simulink model "modelo_kibado_da_mathworks_que_n_funciona"  (R2023a)
settings: Solver=ode45  StartTime=0.0  StopTime=10.0  MaxStep=0.2  RelTol=1e-3
model workspace: external: MATLAB File C:\Users\pinki\OneDrive\aviãozinho\monociclo\numvars.m (data not in the file)
undefined symbols (not defined in the file or in its folder): Ard, Brd, Crd, Drd, K, pos0, vel0
settings Model: Creator=pinki  LastModifiedBy=pinki
settings DataIOCC: InspectSignalLogs=on

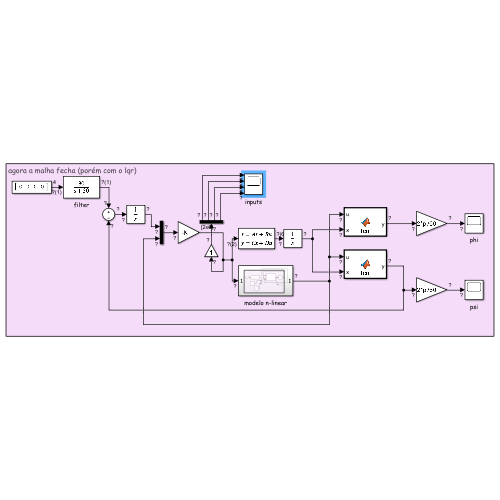
[thumbnail: Simulink's stored preview of the top-level diagram]
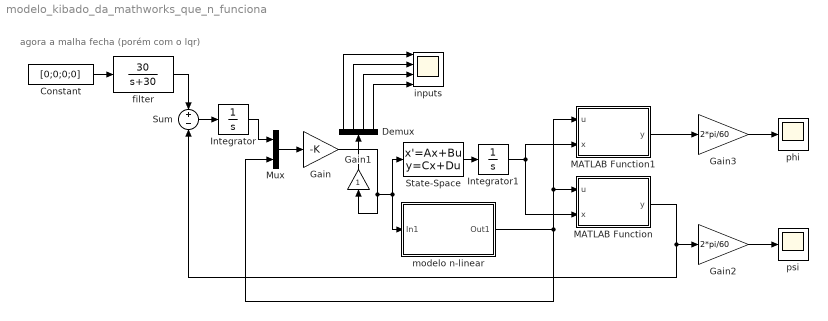
== system modelo_kibado_da_mathworks_que_n_funciona ==
  note: agora a malha fecha (porém com o lqr)
  Constant : Constant  Value=[0;0;0;0]
  Demux : Demux
  Gain : Gain  Gain=-K
  Gain1 : Gain
  Gain2 : Gain  Gain=2*pi/60
  Gain3 : Gain  Gain=2*pi/60
  Integrator : Integrator
  Integrator1 : Integrator
  MATLAB Function : MATLAB Function  TreatAsAtomicUnit=on
  MATLAB Function1 : MATLAB Function  TreatAsAtomicUnit=on
  Mux : Mux  Inputs=2
  State-Space : StateSpace  A=Ard  B=Brd  C=Crd  D=Drd  InitialCondition=0  ContinuousStateAttributes='ss'
  Sum : Sum  Inputs=+-
  filter : TransferFcn  Numerator=[30]  Denominator=[1 30]  ContinuousStateAttributes='filter'
  inputs : Scope  NumInputPorts=4
  modelo n-linear : Subsystem
  phi : Scope
  psi : Scope
  wires:
  filter/1 -> Sum/1
  Sum/1 -> Integrator/1
  Integrator/1 -> Mux/1
  Mux/1 -> Gain/1
  Gain/1 -> modelo n-linear/1(In1), State-Space/1, Gain1/1
  Gain1/1 -> Demux/1
  Demux/1 -> inputs/1
  Demux/2 -> inputs/2
  Demux/3 -> inputs/3
  Demux/4 -> inputs/4
  modelo n-linear/1(Out1) -> MATLAB Function1/1(u), MATLAB Function/1(u), Mux/2
  MATLAB Function/1(y) -> Gain2/1, Sum/2
  Gain2/1 -> psi/1
  MATLAB Function1/1(y) -> Gain3/1
  Gain3/1 -> phi/1
  Constant/1 -> filter/1
  State-Space/1 -> Integrator1/1
  Integrator1/1 -> MATLAB Function/2(x), MATLAB Function1/2(x)

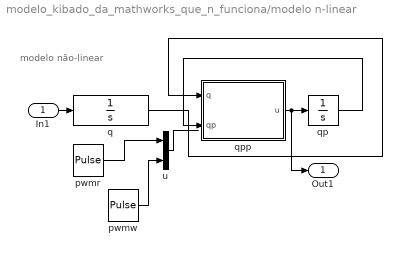
== system modelo_kibado_da_mathworks_que_n_funciona/modelo n-linear ==
  note: modelo não-linear
  In1 : Inport
  pwmr : DiscretePulseGenerator  PulseType=Time based  Amplitude=12  Period=1  PulseWidth=5
  pwmw : DiscretePulseGenerator  PulseType=Time based  Amplitude=12  Period=1  PulseWidth=5
  q : Integrator  InitialCondition=pos0  ContinuousStateAttributes='q'
  qp : Integrator  InitialCondition=vel0  ContinuousStateAttributes='qp'
  qpp : MATLAB Function  Description=nonlinear model  TreatAsAtomicUnit=on
  u : Mux  Inputs=2
  Out1 : Outport
  wires:
  q/1 -> qpp/1(q)
  u/1 -> ?
  qp/1 -> qpp/2(qp)
  pwmw/1 -> u/2
  qpp/1(u) -> Out1/1, qp/1
  pwmr/1 -> u/1
  In1/1 -> q/1

== matlab function modelo_kibado_da_mathworks_que_n_funciona/MATLAB Function ==
  data: u input; y output; x input
function y = fcn(u,x)
y = C*x+ D*u;

== matlab function modelo_kibado_da_mathworks_que_n_funciona/modelo n-linear/qpp ==
  data: q input; qp input; u output
function u = fcn(q,qp)
mono = monociclo;

psi = q(4);
psip = qp(4);

phi = q(2);
phip = qp(2);

thetar = q(1);
thetarp = qp(1);

thetaw = q(3);
thetawp = qp(4);

m11 = mono.jr;
m12 = m11;
m21 = m11;
m22 = (mono.jbw+mono.jr+(mono.mb+mono.mr+mono.mw)*mono.rw^2 ...
+2*(mono.l*(mono.mb*mono.rw+mono.mr*mono.rw)+mono.mr*mono.rw*mono.d)*cos(psi)...
+(mono.l^2*(mono.mb+mono.mr)+mono.mr*mono.d^2+2*mono.l*mono.mr*mono.d)*cos(psi)^2);
m33 = mono.jw+(mono.mb+mono.mr+mono.mw)*mono.rw^2;
m34 = mono.rw*cos(psi)*(mono.mr*mono.d+mono.l*mono.mb+mono.l*mono.mr);
m43 = m34;
m44 = mono.jbr+mono.mb*mono.l^2+mono.mr*mono.l^2+mono.mr*mono.d^2 ...
    +2*mono.l*mono.mr*mono.d;

M = zeros(4,4);
    M(1,1) = m11;
    M(1,2) = m12;
    M(2,1) = m21;
    M(2,2) = m22;
    M(3,3) = m33;
    M(3,4) = m34;
    M(4,3) = m43;
    M(4,4) = m44;

v1 = (mono.ker*mono.ktr*mono.nr*(mono.nr*thetarp))/mono.rer ...
     - mono.bvr*thetar;
v2 = -(mono.ker*mono.ktr*mono.nr*(mono.nr*thetarp))/mono.rer ...
     - 2*(mono.l*mono.mb+mono.mr*mono.d)*mono.rw*phip*psip*sin(psi) ...
     - (mono.mr*mono.l^2+mono.mb*mono.l^2+mono.mr*mono.d^2+2*mono.l*mono.mr*mono.d)*phip*psip*sin(2*psi) ...
     - mono.bvr*thetar;
v3 = (mono.ker*mono.ktw*mono.nw*(mono.nw*thetawp-psip))/mono.rew ...
    + (mono.l*mono.mb+mono.d*mono.mr+mono.l*mono.mr)*mono.rw*psip^2*sin(psi) ...
    + mono.bvw*thetaw;
v4 = -(mono.ker*mono.ktw*mono.nw*(mono.nw*thetawp-psip))/mono.rew ...
    + (mono.l*mono.mb+mono.d*mono.mr+mono.l*mono.mr)*mono.rw*phip^2*sin(psi) ...
    + (sin(2*psi)*phip^2*((mono.mb*mono.l^2)+(mono.mr*mono.l^2) ...
    + (mono.mr*mono.d^2))/2+mono.l*mono.mr*mono.d)+mono.bvw*thetaw;

V = zeros(4,1);
    V(1) = v1;
    V(2) = v2;
    V(3) = v3;
    V(4) = v4;

g2 = -mono.g*sin(phi)*((mono.mb+mono.mr+mono.mw)*mono.rw+(mono.l*mono.mb ...
    + mono.l*mono.mr + mono.mr*mono.d)*cos(psi));
g4 = -mono.g*cos(phi)*sin(psi)*(mono.mr*mono.d+mono.l*mono.mb+mono.l*mono.mr);

G = zeros(4,1);
    G(2) = g2;
    G(4) = g4;

p11 = (12*mono.ktr*mono.nr)/mono.rr;
p12 = -p11;
p23 = (12*mono.ktw*mono.nw)/mono.rw;
p24 = -p23;

P = zeros(4,2);
    P(1,1) = p11;
    P(2,1) = p12;
    P(3,2) = p23;
    P(4,2) = p24;
    
u = P\(M*deriv(qp)+V+G);

== matlab function modelo_kibado_da_mathworks_que_n_funciona/MATLAB Function1 ==
  data: u input; y output; x input
function y = fcn(u,x)
y = C*x+ D*u;
